simulink model "simRouteA_v4_11"  (R2015a)
settings: Solver=FixedStepDiscrete  StartTime=0.0  StopTime=36000  FixedStep=1  RelTol=1e-3
PreLoadFcn:
  | loadTimetable
StopFcn:
  | postProcess
undefined symbols (not defined in the file or in its folder): setBus1IntergenTime, setBus2IntergenTime, setBus3IntergenTime, setBus4IntergenTime
(part 1 of 7)
settings Model: Creator=nhuynh  LastModifiedBy=nhuynh
settings OptimizationCC: ExpressionDepthLimit=2147483647
settings DebuggingCC: UnderspecifiedInitializationDetection=Classic  MergeDetectMultiDrivingBlocksExec=none  SolverPrmCheckMsg=warning  StateNameClashWarn=warning

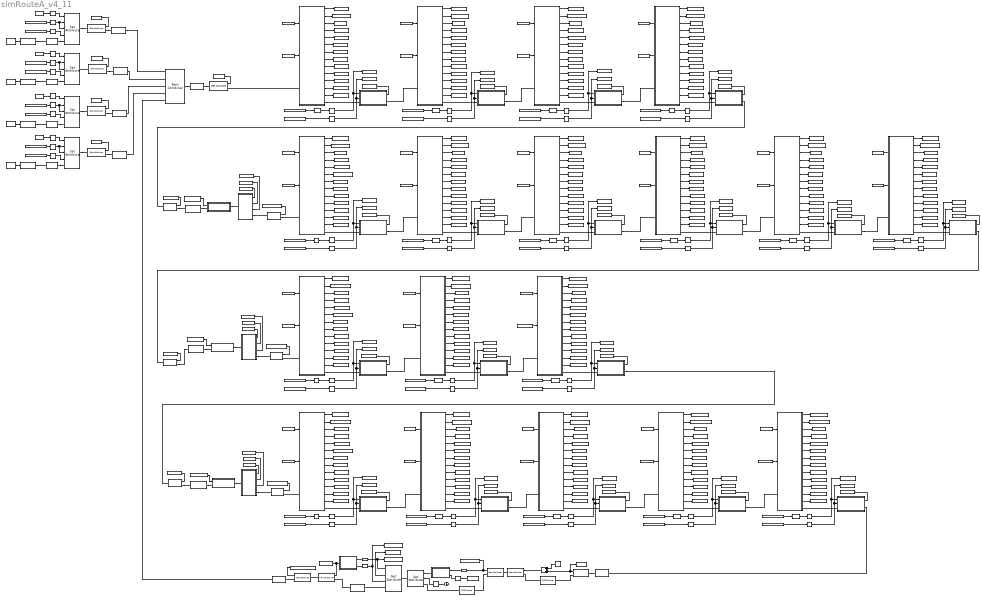
== system simRouteA_v4_11 ==
  Add : Sum
  Clock : Clock
  Constant : Constant
  Constant1 : Constant  Value=20000
  Constant2 : Constant  Value=10000
  Constant3 : Constant  Value=30000
  Constant4 : Constant  Value=40000
  Event Filter : EventFilter  ExecuteSubsystem=Upon sample time hit  SignalEdgeType=Rising
  Event Filter2 : EventFilter  ExecuteSubsystem=Upon sample time hit  SignalEdgeType=Rising
  Event Filter3 : EventFilter  ExecuteSubsystem=Upon sample time hit  SignalEdgeType=Rising
  FIFO Queue{2..6,8,10,13..17} (12 alike) : FIFOQueue
  From Workspace1 : FromWorkspace  VariableName=timetable  Interpolate=off  OutputAfterFinalValue=Holding final value
  From Workspace2 : FromWorkspace  VariableName=timetblChkPnt2  Interpolate=off  OutputAfterFinalValue=Holding final value
  From Workspace3 : FromWorkspace  VariableName=timetblChkPnt3  Interpolate=off  OutputAfterFinalValue=Holding final value
  From Workspace4 : FromWorkspace  VariableName=timetblChkPnt4  Interpolate=off  OutputAfterFinalValue=Holding final value
  Get Attribute{,2,4..8,10..13,17,19,22} (14 alike) : GetAttribute  AttributeName=ID  EvaluatedDefaultAttributeValue={ []}
      settings: OutputPortMap=o1
  Get Attribute3 : GetAttribute  AttributeName=tSched|ID|time  AttributeMissing=Error|Error|Error  AttributeDefaultValue=1|1|1  AttributeTreatAsVector=1|1|1  AttributeSendTiming=After entity departure|After entity departure|After entity departure  EvaluatedDefaultAttributeValue={ []; []; []}
      settings: OutputPortMap=o1,o2,o3
  HoldMultiBus : InfiniteServer  ServiceTimeFrom=Signal port t
  Path Combiner : PathCombiner  NumberInputPorts=5
  Rounding{,1..17} (18 alike) : Rounding  Operator=round
  Set Attribute{,3..5} (4 alike) : SetAttribute  AttributeName=ID|maxCap|vacancy|sec2Brd  AttributeFrom=Signal port|Signal port|Signal port|Signal port  AttributeValue=1|1|1|1  AttributeTreatAsVector=1|1|1|1  EvaluatedAttributeValue={ []; []; []; [] }
      settings: InputPortMap=u0,u1,u2,u3
  Set Attribute8 : SetAttribute  AttributeName=tSched|time  AttributeFrom=Signal port|Signal port  AttributeValue=1|1  AttributeTreatAsVector=1|1  EvaluatedAttributeValue={ []; [] }
      settings: InputPortMap=u0,u1
  Set Attribute9 : SetAttribute  AttributeName=ID  AttributeFrom=Signal port  EvaluatedAttributeValue={ [] }
  Subsystem : Subsystem  TreatAsAtomicUnit=on
      settings: MinAlgLoopOccurrences=on
  Subsystem3 : Subsystem  TreatAsAtomicUnit=on
  T2E{1,4..5,7..10,12..17,19..27,30..31,34..45,48..53,56..59,61..64} (50 alike) : TimedToEventSignal
  atStopS1 : Subsystem
  atStopS10 : Subsystem
  atStopS11 : Subsystem
  atStopS12 : Subsystem
  atStopS13 : Subsystem
  atStopS14 : Subsystem
  atStopS15 : Subsystem
  atStopS16 : Subsystem
  atStopS17 : Subsystem
  atStopS18 : Subsystem
  atStopS2 : Subsystem
  atStopS3 : Subsystem
  atStopS4 : Subsystem
  atStopS5 : Subsystem
  atStopS6 : Subsystem
  atStopS7 : Subsystem
  atStopS8 : Subsystem
  atStopS9 : Subsystem
  bus1Generator : TimeBasedEntityGenerator  GenerateEntitiesUpon=Intergeneration time from port t  GenerateEntityAtSimulationStart=off
  bus1IntergenTime : EventBasedSequence  VectorOutputValues=setBus1IntergenTime()  FormOutputOpt=Setting to infinity
  bus2Generator : TimeBasedEntityGenerator  GenerateEntitiesUpon=Intergeneration time from port t  GenerateEntityAtSimulationStart=off
  bus2IntergenTime : EventBasedSequence  VectorOutputValues=setBus2IntergenTime()  FormOutputOpt=Setting to infinity
  bus3Generator : TimeBasedEntityGenerator  GenerateEntitiesUpon=Intergeneration time from port t  GenerateEntityAtSimulationStart=off
  bus3IntergenTime : EventBasedSequence  VectorOutputValues=setBus3IntergenTime()  FormOutputOpt=Setting to infinity
  bus4Generator : TimeBasedEntityGenerator  GenerateEntitiesUpon=Intergeneration time from port t  GenerateEntityAtSimulationStart=off
  bus4IntergenTime : EventBasedSequence  VectorOutputValues=setBus4IntergenTime()  FormOutputOpt=Setting to infinity
  busIDOut : ToWorkspace  VariableName=busIDOut  SaveFormat=Structure With Time  SampleTime=-1
  chkSchedTimeNormalBusAtCP2 : Subsystem
  chkSchedTimeNormalBusAtCP3 : Subsystem
  chkSchedTimeNormalBusAtCP4 : Subsystem
  delayL1 : FromWorkspace  VariableName=[tLinkDelay,delayL1]  SampleTime=0  OutputAfterFinalValue=Setting to zero
  delayL10 : FromWorkspace  VariableName=[tLinkDelay,delayL10]  SampleTime=0  OutputAfterFinalValue=Setting to zero
  delayL11 : FromWorkspace  VariableName=[tLinkDelay,delayL11]  SampleTime=0  OutputAfterFinalValue=Setting to zero
  delayL12 : FromWorkspace  VariableName=[tLinkDelay,delayL12]  SampleTime=0  OutputAfterFinalValue=Setting to zero
  delayL13 : FromWorkspace  VariableName=[tLinkDelay,delayL13]  SampleTime=0  OutputAfterFinalValue=Setting to zero
  delayL14 : FromWorkspace  VariableName=[tLinkDelay,delayL14]  SampleTime=0  OutputAfterFinalValue=Setting to zero
  delayL15 : FromWorkspace  VariableName=[tLinkDelay,delayL15]  SampleTime=0  OutputAfterFinalValue=Setting to zero
  delayL16 : FromWorkspace  VariableName=[tLinkDelay,delayL16]  SampleTime=0  OutputAfterFinalValue=Setting to zero
  delayL17 : FromWorkspace  VariableName=[tLinkDelay,delayL17]  SampleTime=0  OutputAfterFinalValue=Setting to zero
  delayL18 : FromWorkspace  VariableName=[tLinkDelay,delayL18]  SampleTime=0  OutputAfterFinalValue=Setting to zero
  delayL2 : FromWorkspace  VariableName=[tLinkDelay,delayL2]  SampleTime=0  OutputAfterFinalValue=Setting to zero
  delayL3 : FromWorkspace  VariableName=[tLinkDelay,delayL3]  SampleTime=0  OutputAfterFinalValue=Setting to zero
  delayL4 : FromWorkspace  VariableName=[tLinkDelay,delayL4]  SampleTime=0  OutputAfterFinalValue=Setting to zero
  delayL5 : FromWorkspace  VariableName=[tLinkDelay,delayL5]  SampleTime=0  OutputAfterFinalValue=Setting to zero
  delayL6 : FromWorkspace  VariableName=[tLinkDelay,delayL6]  SampleTime=0  OutputAfterFinalValue=Setting to zero
  delayL7 : FromWorkspace  VariableName=[tLinkDelay,delayL7]  SampleTime=0  OutputAfterFinalValue=Setting to zero
  delayL8 : FromWorkspace  VariableName=[tLinkDelay,delayL8]  SampleTime=0  OutputAfterFinalValue=Setting to zero
  delayL9 : FromWorkspace  VariableName=[tLinkDelay,delayL9]  SampleTime=0  OutputAfterFinalValue=Setting to zero
  dummy Server{,1..3} (4 alike) : SingleServer  ServiceTime=0
  dummyServer : SingleServer  ServiceTime=0
  holdBusAtCP2 : Subsystem
  holdBusAtCP3 : Subsystem
  holdBusAtCP4 : Subsystem
  idAfterCycle : ToWorkspace  VariableName=idAfterCycle  SaveFormat=Structure With Time  SampleTime=-1
  idB4CP2 : ToWorkspace  VariableName=idB4CP2  SaveFormat=Structure With Time  SampleTime=-1
  idB4CP3 : ToWorkspace  VariableName=idB4CP3  SaveFormat=Structure With Time  SampleTime=-1
  idB4CP4 : ToWorkspace  VariableName=idB4CP4  SaveFormat=Structure With Time  SampleTime=-1
  idBus1SA : ToWorkspace  VariableName=idBus1SA  SaveFormat=Structure With Time  SampleTime=-1
  idBus2SA : ToWorkspace  VariableName=idBus2SA  SaveFormat=Structure With Time  SampleTime=-1
  idBus3SA : ToWorkspace  VariableName=idBus3SA  SaveFormat=Structure With Time  SampleTime=-1
  idBus4SA : ToWorkspace  VariableName=idBus4SA  SaveFormat=Structure With Time  SampleTime=-1
  idBusArrAfterCPS11 : ToWorkspace  VariableName=idBusArrAfterCPS11  SaveFormat=Structure With Time  SampleTime=-1
  idBusArrAfterCPS14 : ToWorkspace  VariableName=idBusArrAfterCPS14  SaveFormat=Structure With Time  SampleTime=-1
  idBusArrAfterCPS5 : ToWorkspace  VariableName=idBusArrAfterCPS5  SaveFormat=Structure With Time  SampleTime=-1
  idBusArrS1 : ToWorkspace  VariableName=idBusArrS1  SaveFormat=Structure With Time  SampleTime=-1
  idBusArrS10 : ToWorkspace  VariableName=idBusArrS10  SaveFormat=Structure With Time  SampleTime=-1
  idBusArrS11 : ToWorkspace  VariableName=idBusArrS11  SaveFormat=Structure With Time  SampleTime=-1
  idBusArrS12 : ToWorkspace  VariableName=idBusArrS12  SaveFormat=Structure With Time  SampleTime=-1
  idBusArrS13 : ToWorkspace  VariableName=idBusArrS13  SaveFormat=Structure With Time  SampleTime=-1
  idBusArrS14 : ToWorkspace  VariableName=idBusArrS14  SaveFormat=Structure With Time  SampleTime=-1
  idBusArrS15 : ToWorkspace  VariableName=idBusArrS15  SaveFormat=Structure With Time  SampleTime=-1
  idBusArrS16 : ToWorkspace  VariableName=idBusArrS16  SaveFormat=Structure With Time  SampleTime=-1
  idBusArrS17 : ToWorkspace  VariableName=idBusArrS17  SaveFormat=Structure With Time  SampleTime=-1
  idBusArrS18 : ToWorkspace  VariableName=idBusArrS18  SaveFormat=Structure With Time  SampleTime=-1
  idBusArrS2 : ToWorkspace  VariableName=idBusArrS2  SaveFormat=Structure With Time  SampleTime=-1
  idBusArrS3 : ToWorkspace  VariableName=idBusArrS3  SaveFormat=Structure With Time  SampleTime=-1
  idBusArrS4 : ToWorkspace  VariableName=idBusArrS4  SaveFormat=Structure With Time  SampleTime=-1
  idBusArrS5 : ToWorkspace  VariableName=idBusArrS5  SaveFormat=Structure With Time  SampleTime=-1
  idBusArrS6 : ToWorkspace  VariableName=idBusArrS6  SaveFormat=Structure With Time  SampleTime=-1
  idBusArrS7 : ToWorkspace  VariableName=idBusArrS7  SaveFormat=Structure With Time  SampleTime=-1
  idBusArrS8 : ToWorkspace  VariableName=idBusArrS8  SaveFormat=Structure With Time  SampleTime=-1
  idBusArrS9 : ToWorkspace  VariableName=idBusArrS9  SaveFormat=Structure With Time  SampleTime=-1
  idBusOutChkPntEndCycle : ToWorkspace  VariableName=idBusOutChkPntEndCycle  SaveFormat=Structure With Time  SampleTime=-1
  idBusOutChkPntS11 : ToWorkspace  VariableName=idBusOutChkPntS11  SaveFormat=Structure With Time  SampleTime=-1
  idBusOutChkPntS14 : ToWorkspace  VariableName=idBusOutChkPntS14  SaveFormat=Structure With Time  SampleTime=-1
  idBusOutChkPntS5 : ToWorkspace  VariableName=idBusOutChkPntS5  SaveFormat=Structure With Time  SampleTime=-1
  idBusOutL1 : ToWorkspace  VariableName=idBusOutL1  SaveFormat=Structure With Time  SampleTime=-1
  idBusOutL10 : ToWorkspace  VariableName=idBusOutL10  SaveFormat=Structure With Time  SampleTime=-1
  idBusOutL11 : ToWorkspace  VariableName=idBusOutL11  SaveFormat=Structure With Time  SampleTime=-1
  idBusOutL12 : ToWorkspace  VariableName=idBusOutL12  SaveFormat=Structure With Time  SampleTime=-1
  idBusOutL13 : ToWorkspace  VariableName=idBusOutL13  SaveFormat=Structure With Time  SampleTime=-1
  idBusOutL14 : ToWorkspace  VariableName=idBusOutL14  SaveFormat=Structure With Time  SampleTime=-1
  idBusOutL15 : ToWorkspace  VariableName=idBusOutL15  SaveFormat=Structure With Time  SampleTime=-1
  idBusOutL16 : ToWorkspace  VariableName=idBusOutL16  SaveFormat=Structure With Time  SampleTime=-1
  idBusOutL17 : ToWorkspace  VariableName=idBusOutL17  SaveFormat=Structure With Time  SampleTime=-1
  idBusOutL18 : ToWorkspace  VariableName=idBusOutL18  SaveFormat=Structure With Time  SampleTime=-1
  idBusOutL2 : ToWorkspace  VariableName=idBusOutL2  SaveFormat=Structure With Time  SampleTime=-1
  idBusOutL3 : ToWorkspace  VariableName=idBusOutL3  SaveFormat=Structure With Time  SampleTime=-1
  idBusOutL4 : ToWorkspace  VariableName=idBusOutL4  SaveFormat=Structure With Time  SampleTime=-1
  idBusOutL5 : ToWorkspace  VariableName=idBusOutL5  SaveFormat=Structure With Time  SampleTime=-1
  idBusOutL6 : ToWorkspace  VariableName=idBusOutL6  SaveFormat=Structure With Time  SampleTime=-1
  idBusOutL7 : ToWorkspace  VariableName=idBusOutL7  SaveFormat=Structure With Time  SampleTime=-1
  idBusOutL8 : ToWorkspace  VariableName=idBusOutL8  SaveFormat=Structure With Time  SampleTime=-1
  idBusOutL9 : ToWorkspace  VariableName=idBusOutL9  SaveFormat=Structure With Time  SampleTime=-1
  idBusOutS1 : ToWorkspace  VariableName=idBusOutS1  SaveFormat=Structure With Time  SampleTime=-1
  idBusOutS10 : ToWorkspace  VariableName=idBusOutS10  SaveFormat=Structure With Time  SampleTime=-1
  idBusOutS11 : ToWorkspace  VariableName=idBusOutS11  SaveFormat=Structure With Time  SampleTime=-1
  idBusOutS12 : ToWorkspace  VariableName=idBusOutS12  SaveFormat=Structure With Time  SampleTime=-1
  idBusOutS13 : ToWorkspace  VariableName=idBusOutS13  SaveFormat=Structure With Time  SampleTime=-1
  idBusOutS14 : ToWorkspace  VariableName=idBusOutS14  SaveFormat=Structure With Time  SampleTime=-1
  idBusOutS15 : ToWorkspace  VariableName=idBusOutS15  SaveFormat=Structure With Time  SampleTime=-1
  idBusOutS16 : ToWorkspace  VariableName=idBusOutS16  SaveFormat=Structure With Time  SampleTime=-1
  idBusOutS17 : ToWorkspace  VariableName=idBusOutS17  SaveFormat=Structure With Time  SampleTime=-1
  idBusOutS18 : ToWorkspace  VariableName=idBusOutS18  SaveFormat=Structure With Time  SampleTime=-1
  idBusOutS2 : ToWorkspace  VariableName=idBusOutS2  SaveFormat=Structure With Time  SampleTime=-1
  idBusOutS3 : ToWorkspace  VariableName=idBusOutS3  SaveFormat=Structure With Time  SampleTime=-1
  idBusOutS4 : ToWorkspace  VariableName=idBusOutS4  SaveFormat=Structure With Time  SampleTime=-1
  idBusOutS5 : ToWorkspace  VariableName=idBusOutS5  SaveFormat=Structure With Time  SampleTime=-1
  idBusOutS6 : ToWorkspace  VariableName=idBusOutS6  SaveFormat=Structure With Time  SampleTime=-1
  idBusOutS7 : ToWorkspace  VariableName=idBusOutS7  SaveFormat=Structure With Time  SampleTime=-1
  idBusOutS8 : ToWorkspace  VariableName=idBusOutS8  SaveFormat=Structure With Time  SampleTime=-1
  idBusOutS9 : ToWorkspace  VariableName=idBusOutS9  SaveFormat=Structure With Time  SampleTime=-1
  idInit : ToWorkspace  VariableName=idInit  SaveFormat=Structure With Time  SampleTime=-1
  idNxtNormalBus : ToWorkspace  VariableName=idNxtNormalBus  SaveFormat=Structure With Time  SampleTime=-1
  inTransitLinkL1 : Subsystem
  inTransitLinkL10 : Subsystem
  inTransitLinkL11 : Subsystem
  inTransitLinkL12 : Subsystem
  inTransitLinkL13 : Subsystem
  inTransitLinkL14 : Subsystem
  inTransitLinkL15 : Subsystem
  inTransitLinkL16 : Subsystem
  inTransitLinkL17 : Subsystem
  inTransitLinkL18 : Subsystem
  inTransitLinkL2 : Subsystem
  inTransitLinkL3 : Subsystem
  inTransitLinkL4 : Subsystem
  inTransitLinkL5 : Subsystem
  inTransitLinkL6 : Subsystem
  inTransitLinkL7 : Subsystem
  inTransitLinkL8 : Subsystem
  inTransitLinkL9 : Subsystem
  intgPaxAlightS1 : ToWorkspace  VariableName=paxAlightIntS1  SaveFormat=Structure With Time  SampleTime=-1
  intgPaxAlightS10 : ToWorkspace  VariableName=paxAlightIntS10  SaveFormat=Structure With Time  SampleTime=-1
  intgPaxAlightS11 : ToWorkspace  VariableName=paxAlightIntS11  SaveFormat=Structure With Time  SampleTime=-1
  intgPaxAlightS12 : ToWorkspace  VariableName=paxAlightIntS12  SaveFormat=Structure With Time  SampleTime=-1
  intgPaxAlightS13 : ToWorkspace  VariableName=paxAlightIntS13  SaveFormat=Structure With Time  SampleTime=-1
  intgPaxAlightS14 : ToWorkspace  VariableName=paxAlightIntS14  SaveFormat=Structure With Time  SampleTime=-1
  intgPaxAlightS15 : ToWorkspace  VariableName=paxAlightIntS15  SaveFormat=Structure With Time  SampleTime=-1
  intgPaxAlightS16 : ToWorkspace  VariableName=paxAlightIntS16  SaveFormat=Structure With Time  SampleTime=-1
  intgPaxAlightS17 : ToWorkspace  VariableName=paxAlightIntS17  SaveFormat=Structure With Time  SampleTime=-1
  intgPaxAlightS18 : ToWorkspace  VariableName=paxAlightIntS18  SaveFormat=Structure With Time  SampleTime=-1
  intgPaxAlightS2 : ToWorkspace  VariableName=paxAlightIntS2  SaveFormat=Structure With Time  SampleTime=-1
  intgPaxAlightS3 : ToWorkspace  VariableName=paxAlightIntS3  SaveFormat=Structure With Time  SampleTime=-1
  intgPaxAlightS4 : ToWorkspace  VariableName=paxAlightIntS4  SaveFormat=Structure With Time  SampleTime=-1
  intgPaxAlightS5 : ToWorkspace  VariableName=paxAlightIntS5  SaveFormat=Structure With Time  SampleTime=-1
  intgPaxAlightS6 : ToWorkspace  VariableName=paxAlightIntS6  SaveFormat=Structure With Time  SampleTime=-1
  intgPaxAlightS7 : ToWorkspace  VariableName=paxAlightIntS7  SaveFormat=Structure With Time  SampleTime=-1
  intgPaxAlightS8 : ToWorkspace  VariableName=paxAlightIntS8  SaveFormat=Structure With Time  SampleTime=-1
  intgPaxAlightS9 : ToWorkspace  VariableName=paxAlightIntS9  SaveFormat=Structure With Time  SampleTime=-1
  intgPaxArrS1 : ToWorkspace  VariableName=paxArrIntS1  SaveFormat=Structure With Time  SampleTime=-1
  intgPaxArrS10 : ToWorkspace  VariableName=paxArrIntS10  SaveFormat=Structure With Time  SampleTime=-1
  intgPaxArrS11 : ToWorkspace  VariableName=paxArrIntS11  SaveFormat=Structure With Time  SampleTime=-1
  intgPaxArrS12 : ToWorkspace  VariableName=paxArrIntS12  SaveFormat=Structure With Time  SampleTime=-1
  intgPaxArrS13 : ToWorkspace  VariableName=paxArrIntS13  SaveFormat=Structure With Time  SampleTime=-1
  intgPaxArrS14 : ToWorkspace  VariableName=paxArrIntS14  SaveFormat=Structure With Time  SampleTime=-1
  intgPaxArrS15 : ToWorkspace  VariableName=paxArrIntS15  SaveFormat=Structure With Time  SampleTime=-1
  intgPaxArrS16 : ToWorkspace  VariableName=paxArrIntS16  SaveFormat=Structure With Time  SampleTime=-1
  intgPaxArrS17 : ToWorkspace  VariableName=paxArrIntS17  SaveFormat=Structure With Time  SampleTime=-1
  intgPaxArrS18 : ToWorkspace  VariableName=paxArrIntS18  SaveFormat=Structure With Time  SampleTime=-1
  intgPaxArrS2 : ToWorkspace  VariableName=paxArrIntS2  SaveFormat=Structure With Time  SampleTime=-1
  intgPaxArrS3 : ToWorkspace  VariableName=paxArrIntS3  SaveFormat=Structure With Time  SampleTime=-1
  intgPaxArrS4 : ToWorkspace  VariableName=paxArrIntS4  SaveFormat=Structure With Time  SampleTime=-1
  intgPaxArrS5 : ToWorkspace  VariableName=paxArrIntS5  SaveFormat=Structure With Time  SampleTime=-1
  intgPaxArrS6 : ToWorkspace  VariableName=paxArrIntS6  SaveFormat=Structure With Time  SampleTime=-1
  intgPaxArrS7 : ToWorkspace  VariableName=paxArrIntS7  SaveFormat=Structure With Time  SampleTime=-1
  intgPaxArrS8 : ToWorkspace  VariableName=paxArrIntS8  SaveFormat=Structure With Time  SampleTime=-1
  intgPaxArrS9 : ToWorkspace  VariableName=paxArrIntS9  SaveFormat=Structure With Time  SampleTime=-1
  maxCapBus{1..4} (4 alike) : FromWorkspace  VariableName=[tConst,maxBusCap]  SampleTime=0  OutputAfterFinalValue=Holding final value
  newVacanS1 : ToWorkspace  VariableName=newVacanS1  SaveFormat=Structure With Time  SampleTime=-1
  newVacanS10 : ToWorkspace  VariableName=newVacanS10  SaveFormat=Structure With Time  SampleTime=-1
  newVacanS11 : ToWorkspace  VariableName=newVacanS11  SaveFormat=Structure With Time  SampleTime=-1
  newVacanS12 : ToWorkspace  VariableName=newVacanS12  SaveFormat=Structure With Time  SampleTime=-1
  newVacanS13 : ToWorkspace  VariableName=newVacanS13  SaveFormat=Structure With Time  SampleTime=-1
  newVacanS14 : ToWorkspace  VariableName=newVacanS14  SaveFormat=Structure With Time  SampleTime=-1
  newVacanS15 : ToWorkspace  VariableName=newVacanS15  SaveFormat=Structure With Time  SampleTime=-1
  newVacanS16 : ToWorkspace  VariableName=newVacanS16  SaveFormat=Structure With Time  SampleTime=-1
  newVacanS17 : ToWorkspace  VariableName=newVacanS17  SaveFormat=Structure With Time  SampleTime=-1
  newVacanS18 : ToWorkspace  VariableName=newVacanS18  SaveFormat=Structure With Time  SampleTime=-1
  newVacanS2 : ToWorkspace  VariableName=newVacanS2  SaveFormat=Structure With Time  SampleTime=-1
  newVacanS3 : ToWorkspace  VariableName=newVacanS3  SaveFormat=Structure With Time  SampleTime=-1
  newVacanS4 : ToWorkspace  VariableName=newVacanS4  SaveFormat=Structure With Time  SampleTime=-1
  newVacanS5 : ToWorkspace  VariableName=newVacanS5  SaveFormat=Structure With Time  SampleTime=-1
  newVacanS6 : ToWorkspace  VariableName=newVacanS6  SaveFormat=Structure With Time  SampleTime=-1
  newVacanS7 : ToWorkspace  VariableName=newVacanS7  SaveFormat=Structure With Time  SampleTime=-1
  newVacanS8 : ToWorkspace  VariableName=newVacanS8  SaveFormat=Structure With Time  SampleTime=-1
  newVacanS9 : ToWorkspace  VariableName=newVacanS9  SaveFormat=Structure With Time  SampleTime=-1
  paxAlightS1 : ToWorkspace  VariableName=paxAlightS1  SaveFormat=Structure With Time  SampleTime=-1
  paxAlightS10 : ToWorkspace  VariableName=paxAlightS10  SaveFormat=Structure With Time  SampleTime=-1
  paxAlightS11 : ToWorkspace  VariableName=paxAlightS11  SaveFormat=Structure With Time  SampleTime=-1
  paxAlightS12 : ToWorkspace  VariableName=paxAlightS12  SaveFormat=Structure With Time  SampleTime=-1
  paxAlightS13 : ToWorkspace  VariableName=paxAlightS13  SaveFormat=Structure With Time  SampleTime=-1
  paxAlightS14 : ToWorkspace  VariableName=paxAlightS14  SaveFormat=Structure With Time  SampleTime=-1
  paxAlightS15 : ToWorkspace  VariableName=paxAlightS15  SaveFormat=Structure With Time  SampleTime=-1
  paxAlightS16 : ToWorkspace  VariableName=paxAlightS16  SaveFormat=Structure With Time  SampleTime=-1
  paxAlightS17 : ToWorkspace  VariableName=paxAlightS17  SaveFormat=Structure With Time  SampleTime=-1
  paxAlightS18 : ToWorkspace  VariableName=paxAlightS18  SaveFormat=Structure With Time  SampleTime=-1
  paxAlightS2 : ToWorkspace  VariableName=paxAlightS2  SaveFormat=Structure With Time  SampleTime=-1
  paxAlightS3 : ToWorkspace  VariableName=paxAlightS3  SaveFormat=Structure With Time  SampleTime=-1
  paxAlightS4 : ToWorkspace  VariableName=paxAlightS4  SaveFormat=Structure With Time  SampleTime=-1
  paxAlightS5 : ToWorkspace  VariableName=paxAlightS5  SaveFormat=Structure With Time  SampleTime=-1
  paxAlightS6 : ToWorkspace  VariableName=paxAlightS6  SaveFormat=Structure With Time  SampleTime=-1
  paxAlightS7 : ToWorkspace  VariableName=paxAlightS7  SaveFormat=Structure With Time  SampleTime=-1
  paxAlightS8 : ToWorkspace  VariableName=paxAlightS8  SaveFormat=Structure With Time  SampleTime=-1
  paxAlightS9 : ToWorkspace  VariableName=paxAlightS9  SaveFormat=Structure With Time  SampleTime=-1
  paxBoardS1 : ToWorkspace  VariableName=paxBoardS1  SaveFormat=Structure With Time  SampleTime=-1
  paxBoardS10 : ToWorkspace  VariableName=paxBoardS10  SaveFormat=Structure With Time  SampleTime=-1
  paxBoardS11 : ToWorkspace  VariableName=paxBoardS11  SaveFormat=Structure With Time  SampleTime=-1
  paxBoardS12 : ToWorkspace  VariableName=paxBoardS12  SaveFormat=Structure With Time  SampleTime=-1
  paxBoardS13 : ToWorkspace  VariableName=paxBoardS13  SaveFormat=Structure With Time  SampleTime=-1
  paxBoardS14 : ToWorkspace  VariableName=paxBoardS14  SaveFormat=Structure With Time  SampleTime=-1
  paxBoardS15 : ToWorkspace  VariableName=paxBoardS15  SaveFormat=Structure With Time  SampleTime=-1
  paxBoardS16 : ToWorkspace  VariableName=paxBoardS16  SaveFormat=Structure With Time  SampleTime=-1
  paxBoardS17 : ToWorkspace  VariableName=paxBoardS17  SaveFormat=Structure With Time  SampleTime=-1
  paxBoardS18 : ToWorkspace  VariableName=paxBoardS18  SaveFormat=Structure With Time  SampleTime=-1
  paxBoardS2 : ToWorkspace  VariableName=paxBoardS2  SaveFormat=Structure With Time  SampleTime=-1
  paxBoardS3 : ToWorkspace  VariableName=paxBoardS3  SaveFormat=Structure With Time  SampleTime=-1
  paxBoardS4 : ToWorkspace  VariableName=paxBoardS4  SaveFormat=Structure With Time  SampleTime=-1
  paxBoardS5 : ToWorkspace  VariableName=paxBoardS5  SaveFormat=Structure With Time  SampleTime=-1
  paxBoardS6 : ToWorkspace  VariableName=paxBoardS6  SaveFormat=Structure With Time  SampleTime=-1
  paxBoardS7 : ToWorkspace  VariableName=paxBoardS7  SaveFormat=Structure With Time  SampleTime=-1
  paxBoardS8 : ToWorkspace  VariableName=paxBoardS8  SaveFormat=Structure With Time  SampleTime=-1
  paxBoardS9 : ToWorkspace  VariableName=paxBoardS9  SaveFormat=Structure With Time  SampleTime=-1
  paxDemandS1 : ToWorkspace  VariableName=paxDemandS1  SaveFormat=Structure With Time  SampleTime=-1
  paxDemandS10 : ToWorkspace  VariableName=paxDemandS10  SaveFormat=Structure With Time  SampleTime=-1
  paxDemandS11 : ToWorkspace  VariableName=paxDemandS11  SaveFormat=Structure With Time  SampleTime=-1
  paxDemandS12 : ToWorkspace  VariableName=paxDemandS12  SaveFormat=Structure With Time  SampleTime=-1
  paxDemandS13 : ToWorkspace  VariableName=paxDemandS13  SaveFormat=Structure With Time  SampleTime=-1
  paxDemandS14 : ToWorkspace  VariableName=paxDemandS14  SaveFormat=Structure With Time  SampleTime=-1
  paxDemandS15 : ToWorkspace  VariableName=paxDemandS15  SaveFormat=Structure With Time  SampleTime=-1
  paxDemandS16 : ToWorkspace  VariableName=paxDemandS16  SaveFormat=Structure With Time  SampleTime=-1
  paxDemandS17 : ToWorkspace  VariableName=paxDemandS17  SaveFormat=Structure With Time  SampleTime=-1
  paxDemandS18 : ToWorkspace  VariableName=paxDemandS18  SaveFormat=Structure With Time  SampleTime=-1
  paxDemandS2 : ToWorkspace  VariableName=paxDemandS2  SaveFormat=Structure With Time  SampleTime=-1
  paxDemandS3 : ToWorkspace  VariableName=paxDemandS3  SaveFormat=Structure With Time  SampleTime=-1
  paxDemandS4 : ToWorkspace  VariableName=paxDemandS4  SaveFormat=Structure With Time  SampleTime=-1
  paxDemandS5 : ToWorkspace  VariableName=paxDemandS5  SaveFormat=Structure With Time  SampleTime=-1
  paxDemandS6 : ToWorkspace  VariableName=paxDemandS6  SaveFormat=Structure With Time  SampleTime=-1
  paxDemandS7 : ToWorkspace  VariableName=paxDemandS7  SaveFormat=Structure With Time  SampleTime=-1
  paxDemandS8 : ToWorkspace  VariableName=paxDemandS8  SaveFormat=Structure With Time  SampleTime=-1
  paxDemandS9 : ToWorkspace  VariableName=paxDemandS9  SaveFormat=Structure With Time  SampleTime=-1
  paxRemainS1 : ToWorkspace  VariableName=paxRemainS1  SaveFormat=Structure With Time  SampleTime=-1
  paxRemainS10 : ToWorkspace  VariableName=paxRemainS10  SaveFormat=Structure With Time  SampleTime=-1
  paxRemainS11 : ToWorkspace  VariableName=paxRemainS11  SaveFormat=Structure With Time  SampleTime=-1
  paxRemainS12 : ToWorkspace  VariableName=paxRemainS12  SaveFormat=Structure With Time  SampleTime=-1
  paxRemainS13 : ToWorkspace  VariableName=paxRemainS13  SaveFormat=Structure With Time  SampleTime=-1
  paxRemainS14 : ToWorkspace  VariableName=paxRemainS14  SaveFormat=Structure With Time  SampleTime=-1
  paxRemainS15 : ToWorkspace  VariableName=paxRemainS15  SaveFormat=Structure With Time  SampleTime=-1
  paxRemainS16 : ToWorkspace  VariableName=paxRemainS16  SaveFormat=Structure With Time  SampleTime=-1
  paxRemainS17 : ToWorkspace  VariableName=paxRemainS17  SaveFormat=Structure With Time  SampleTime=-1
  paxRemainS18 : ToWorkspace  VariableName=paxRemainS18  SaveFormat=Structure With Time  SampleTime=-1
  paxRemainS2 : ToWorkspace  VariableName=paxRemainS2  SaveFormat=Structure With Time  SampleTime=-1
  paxRemainS3 : ToWorkspace  VariableName=paxRemainS3  SaveFormat=Structure With Time  SampleTime=-1
  paxRemainS4 : ToWorkspace  VariableName=paxRemainS4  SaveFormat=Structure With Time  SampleTime=-1
  paxRemainS5 : ToWorkspace  VariableName=paxRemainS5  SaveFormat=Structure With Time  SampleTime=-1
  paxRemainS6 : ToWorkspace  VariableName=paxRemainS6  SaveFormat=Structure With Time  SampleTime=-1
  paxRemainS7 : ToWorkspace  VariableName=paxRemainS7  SaveFormat=Structure With Time  SampleTime=-1
  paxRemainS8 : ToWorkspace  VariableName=paxRemainS8  SaveFormat=Structure With Time  SampleTime=-1
  paxRemainS9 : ToWorkspace  VariableName=paxRemainS9  SaveFormat=Structure With Time  SampleTime=-1
  paxWaitS1 : ToWorkspace  VariableName=paxWaitS1  SaveFormat=Structure With Time  SampleTime=-1
  paxWaitS10 : ToWorkspace  VariableName=paxWaitS10  SaveFormat=Structure With Time  SampleTime=-1
  paxWaitS11 : ToWorkspace  VariableName=paxWaitS11  SaveFormat=Structure With Time  SampleTime=-1
  paxWaitS12 : ToWorkspace  VariableName=paxWaitS12  SaveFormat=Structure With Time  SampleTime=-1
  paxWaitS13 : ToWorkspace  VariableName=paxWaitS13  SaveFormat=Structure With Time  SampleTime=-1
  paxWaitS14 : ToWorkspace  VariableName=paxWaitS14  SaveFormat=Structure With Time  SampleTime=-1
  paxWaitS15 : ToWorkspace  VariableName=paxWaitS15  SaveFormat=Structure With Time  SampleTime=-1
  paxWaitS16 : ToWorkspace  VariableName=paxWaitS16  SaveFormat=Structure With Time  SampleTime=-1
  paxWaitS17 : ToWorkspace  VariableName=paxWaitS17  SaveFormat=Structure With Time  SampleTime=-1
  paxWaitS18 : ToWorkspace  VariableName=paxWaitS18  SaveFormat=Structure With Time  SampleTime=-1
  paxWaitS2 : ToWorkspace  VariableName=paxWaitS2  SaveFormat=Structure With Time  SampleTime=-1
  paxWaitS3 : ToWorkspace  VariableName=paxWaitS3  SaveFormat=Structure With Time  SampleTime=-1
  paxWaitS4 : ToWorkspace  VariableName=paxWaitS4  SaveFormat=Structure With Time  SampleTime=-1
  paxWaitS5 : ToWorkspace  VariableName=paxWaitS5  SaveFormat=Structure With Time  SampleTime=-1
  paxWaitS6 : ToWorkspace  VariableName=paxWaitS6  SaveFormat=Structure With Time  SampleTime=-1
  paxWaitS7 : ToWorkspace  VariableName=paxWaitS7  SaveFormat=Structure With Time  SampleTime=-1
  paxWaitS8 : ToWorkspace  VariableName=paxWaitS8  SaveFormat=Structure With Time  SampleTime=-1
  paxWaitS9 : ToWorkspace  VariableName=paxWaitS9  SaveFormat=Structure With Time  SampleTime=-1
  randDelayL1 : ToWorkspace  VariableName=randDelayL1  SaveFormat=Structure With Time  SampleTime=-1
  randDelayL10 : ToWorkspace  VariableName=randDelayL10  SaveFormat=Structure With Time  SampleTime=-1
  randDelayL11 : ToWorkspace  VariableName=randDelayL11  SaveFormat=Structure With Time  SampleTime=-1
  randDelayL12 : ToWorkspace  VariableName=randDelayL12  SaveFormat=Structure With Time  SampleTime=-1
  randDelayL13 : ToWorkspace  VariableName=randDelayL13  SaveFormat=Structure With Time  SampleTime=-1
  randDelayL14 : ToWorkspace  VariableName=randDelayL14  SaveFormat=Structure With Time  SampleTime=-1
  randDelayL15 : ToWorkspace  VariableName=randDelayL15  SaveFormat=Structure With Time  SampleTime=-1
  randDelayL16 : ToWorkspace  VariableName=randDelayL16  SaveFormat=Structure With Time  SampleTime=-1
  randDelayL17 : ToWorkspace  VariableName=randDelayL17  SaveFormat=Structure With Time  SampleTime=-1
  randDelayL18 : ToWorkspace  VariableName=randDelayL18  SaveFormat=Structure With Time  SampleTime=-1
  randDelayL2 : ToWorkspace  VariableName=randDelayL2  SaveFormat=Structure With Time  SampleTime=-1
  randDelayL3 : ToWorkspace  VariableName=randDelayL3  SaveFormat=Structure With Time  SampleTime=-1
  randDelayL4 : ToWorkspace  VariableName=randDelayL4  SaveFormat=Structure With Time  SampleTime=-1
  randDelayL5 : ToWorkspace  VariableName=randDelayL5  SaveFormat=Structure With Time  SampleTime=-1
  randDelayL6 : ToWorkspace  VariableName=randDelayL6  SaveFormat=Structure With Time  SampleTime=-1
  randDelayL7 : ToWorkspace  VariableName=randDelayL7  SaveFormat=Structure With Time  SampleTime=-1
  randDelayL8 : ToWorkspace  VariableName=randDelayL8  SaveFormat=Structure With Time  SampleTime=-1
  randDelayL9 : ToWorkspace  VariableName=randDelayL9  SaveFormat=Structure With Time  SampleTime=-1
  ratePaxAlightS1 : FromWorkspace  VariableName=[t,alightS1]  SampleTime=0  OutputAfterFinalValue=Setting to zero
  ratePaxAlightS10 : FromWorkspace  VariableName=[t,alightS10]  SampleTime=0  OutputAfterFinalValue=Setting to zero
  ratePaxAlightS11 : FromWorkspace  VariableName=[t,alightS11]  SampleTime=0  OutputAfterFinalValue=Setting to zero
  ratePaxAlightS12 : FromWorkspace  VariableName=[t,alightS12]  SampleTime=0  OutputAfterFinalValue=Setting to zero
  ratePaxAlightS13 : FromWorkspace  VariableName=[t,alightS13]  SampleTime=0  OutputAfterFinalValue=Setting to zero
  ratePaxAlightS14 : FromWorkspace  VariableName=[t,alightS14]  SampleTime=0  OutputAfterFinalValue=Setting to zero
  ratePaxAlightS15 : FromWorkspace  VariableName=[t,alightS15]  SampleTime=0  OutputAfterFinalValue=Setting to zero
  ratePaxAlightS16 : FromWorkspace  VariableName=[t,alightS16]  SampleTime=0  OutputAfterFinalValue=Setting to zero
  ratePaxAlightS17 : FromWorkspace  VariableName=[t,alightS17]  SampleTime=0  OutputAfterFinalValue=Setting to zero
  ratePaxAlightS18 : FromWorkspace  VariableName=[t,alightS18]  SampleTime=0  OutputAfterFinalValue=Setting to zero
  ratePaxAlightS2 : FromWorkspace  VariableName=[t,alightS2]  SampleTime=0  OutputAfterFinalValue=Setting to zero
  ratePaxAlightS3 : FromWorkspace  VariableName=[t,alightS3]  SampleTime=0  OutputAfterFinalValue=Setting to zero
  ratePaxAlightS4 : FromWorkspace  VariableName=[t,alightS4]  SampleTime=0  OutputAfterFinalValue=Setting to zero
  ratePaxAlightS5 : FromWorkspace  VariableName=[t,alightS5]  SampleTime=0  OutputAfterFinalValue=Setting to zero
  ratePaxAlightS6 : FromWorkspace  VariableName=[t,alightS6]  SampleTime=0  OutputAfterFinalValue=Setting to zero
  ratePaxAlightS7 : FromWorkspace  VariableName=[t,alightS7]  SampleTime=0  OutputAfterFinalValue=Setting to zero
  ratePaxAlightS8 : FromWorkspace  VariableName=[t,alightS8]  SampleTime=0  OutputAfterFinalValue=Setting to zero
  ratePaxAlightS9 : FromWorkspace  VariableName=[t,alightS9]  SampleTime=0  OutputAfterFinalValue=Setting to zero
  ratePaxArrS1 : FromWorkspace  VariableName=[t,arrS1]  SampleTime=0  OutputAfterFinalValue=Setting to zero
  ratePaxArrS10 : FromWorkspace  VariableName=[t,arrS10]  SampleTime=0  OutputAfterFinalValue=Setting to zero
  ratePaxArrS11 : FromWorkspace  VariableName=[t,arrS11]  SampleTime=0  OutputAfterFinalValue=Setting to zero
  ratePaxArrS12 : FromWorkspace  VariableName=[t,arrS12]  SampleTime=0  OutputAfterFinalValue=Setting to zero
  ratePaxArrS13 : FromWorkspace  VariableName=[t,arrS13]  SampleTime=0  OutputAfterFinalValue=Setting to zero
  ratePaxArrS14 : FromWorkspace  VariableName=[t,arrS14]  SampleTime=0  OutputAfterFinalValue=Setting to zero
  ratePaxArrS15 : FromWorkspace  VariableName=[t,arrS15]  SampleTime=0  OutputAfterFinalValue=Setting to zero
  ratePaxArrS16 : FromWorkspace  VariableName=[t,arrS16]  SampleTime=0  OutputAfterFinalValue=Setting to zero
  ratePaxArrS17 : FromWorkspace  VariableName=[t,arrS17]  SampleTime=0  OutputAfterFinalValue=Setting to zero
  ratePaxArrS18 : FromWorkspace  VariableName=[t,arrS18]  SampleTime=0  OutputAfterFinalValue=Setting to zero
  ratePaxArrS2 : FromWorkspace  VariableName=[t,arrS2]  SampleTime=0  OutputAfterFinalValue=Setting to zero
  ratePaxArrS3 : FromWorkspace  VariableName=[t,arrS3]  SampleTime=0  OutputAfterFinalValue=Setting to zero
  ratePaxArrS4 : FromWorkspace  VariableName=[t,arrS4]  SampleTime=0  OutputAfterFinalValue=Setting to zero
  ratePaxArrS5 : FromWorkspace  VariableName=[t,arrS5]  SampleTime=0  OutputAfterFinalValue=Setting to zero
  ratePaxArrS6 : FromWorkspace  VariableName=[t,arrS6]  SampleTime=0  OutputAfterFinalValue=Setting to zero
  ratePaxArrS7 : FromWorkspace  VariableName=[t,arrS7]  SampleTime=0  OutputAfterFinalValue=Setting to zero
  ratePaxArrS8 : FromWorkspace  VariableName=[t,arrS8]  SampleTime=0  OutputAfterFinalValue=Setting to zero
  ratePaxArrS9 : FromWorkspace  VariableName=[t,arrS9]  SampleTime=0  OutputAfterFinalValue=Setting to zero
  rawPaxAlightS1 : ToWorkspace  VariableName=rawPaxAlightS1  SaveFormat=Structure With Time  SampleTime=-1
  rawPaxAlightS10 : ToWorkspace  VariableName=rawPaxAlightS10  SaveFormat=Structure With Time  SampleTime=-1
  rawPaxAlightS11 : ToWorkspace  VariableName=rawPaxAlightS11  SaveFormat=Structure With Time  SampleTime=-1
  rawPaxAlightS12 : ToWorkspace  VariableName=rawPaxAlightS12  SaveFormat=Structure With Time  SampleTime=-1
  rawPaxAlightS13 : ToWorkspace  VariableName=rawPaxAlightS13  SaveFormat=Structure With Time  SampleTime=-1
  rawPaxAlightS14 : ToWorkspace  VariableName=rawPaxAlightS14  SaveFormat=Structure With Time  SampleTime=-1
  rawPaxAlightS15 : ToWorkspace  VariableName=rawPaxAlightS15  SaveFormat=Structure With Time  SampleTime=-1
  rawPaxAlightS16 : ToWorkspace  VariableName=rawPaxAlightS16  SaveFormat=Structure With Time  SampleTime=-1
  rawPaxAlightS17 : ToWorkspace  VariableName=rawPaxAlightS17  SaveFormat=Structure With Time  SampleTime=-1
  rawPaxAlightS18 : ToWorkspace  VariableName=rawPaxAlightS18  SaveFormat=Structure With Time  SampleTime=-1
  rawPaxAlightS2 : ToWorkspace  VariableName=rawPaxAlightS2  SaveFormat=Structure With Time  SampleTime=-1
  rawPaxAlightS3 : ToWorkspace  VariableName=rawPaxAlightS3  SaveFormat=Structure With Time  SampleTime=-1
  rawPaxAlightS4 : ToWorkspace  VariableName=rawPaxAlightS4  SaveFormat=Structure With Time  SampleTime=-1
  rawPaxAlightS5 : ToWorkspace  VariableName=rawPaxAlightS5  SaveFormat=Structure With Time  SampleTime=-1
  rawPaxAlightS6 : ToWorkspace  VariableName=rawPaxAlightS6  SaveFormat=Structure With Time  SampleTime=-1
  rawPaxAlightS7 : ToWorkspace  VariableName=rawPaxAlightS7  SaveFormat=Structure With Time  SampleTime=-1
  rawPaxAlightS8 : ToWorkspace  VariableName=rawPaxAlightS8  SaveFormat=Structure With Time  SampleTime=-1
  rawPaxAlightS9 : ToWorkspace  VariableName=rawPaxAlightS9  SaveFormat=Structure With Time  SampleTime=-1
  rawPaxDemandS1 : ToWorkspace  VariableName=rawPaxDemandS1  SaveFormat=Structure With Time  SampleTime=-1
  rawPaxDemandS10 : ToWorkspace  VariableName=rawPaxDemandS10  SaveFormat=Structure With Time  SampleTime=-1
  rawPaxDemandS11 : ToWorkspace  VariableName=rawPaxDemandS11  SaveFormat=Structure With Time  SampleTime=-1
  rawPaxDemandS12 : ToWorkspace  VariableName=rawPaxDemandS12  SaveFormat=Structure With Time  SampleTime=-1
  rawPaxDemandS13 : ToWorkspace  VariableName=rawPaxDemandS13  SaveFormat=Structure With Time  SampleTime=-1
  rawPaxDemandS14 : ToWorkspace  VariableName=rawPaxDemandS14  SaveFormat=Structure With Time  SampleTime=-1
  rawPaxDemandS15 : ToWorkspace  VariableName=rawPaxDemandS15  SaveFormat=Structure With Time  SampleTime=-1
  rawPaxDemandS16 : ToWorkspace  VariableName=rawPaxDemandS16  SaveFormat=Structure With Time  SampleTime=-1
  rawPaxDemandS17 : ToWorkspace  VariableName=rawPaxDemandS17  SaveFormat=Structure With Time  SampleTime=-1
  rawPaxDemandS18 : ToWorkspace  VariableName=rawPaxDemandS18  SaveFormat=Structure With Time  SampleTime=-1
  rawPaxDemandS2 : ToWorkspace  VariableName=rawPaxDemandS2  SaveFormat=Structure With Time  SampleTime=-1
  rawPaxDemandS3 : ToWorkspace  VariableName=rawPaxDemandS3  SaveFormat=Structure With Time  SampleTime=-1
  rawPaxDemandS4 : ToWorkspace  VariableName=rawPaxDemandS4  SaveFormat=Structure With Time  SampleTime=-1
  rawPaxDemandS5 : ToWorkspace  VariableName=rawPaxDemandS5  SaveFormat=Structure With Time  SampleTime=-1
  rawPaxDemandS6 : ToWorkspace  VariableName=rawPaxDemandS6  SaveFormat=Structure With Time  SampleTime=-1
  rawPaxDemandS7 : ToWorkspace  VariableName=rawPaxDemandS7  SaveFormat=Structure With Time  SampleTime=-1
  rawPaxDemandS8 : ToWorkspace  VariableName=rawPaxDemandS8  SaveFormat=Structure With Time  SampleTime=-1
  rawPaxDemandS9 : ToWorkspace  VariableName=rawPaxDemandS9  SaveFormat=Structure With Time  SampleTime=-1
  tBoardPerPax{,1..3} (4 alike) : FromWorkspace  VariableName=[tConst,tBoardPerPax]  SampleTime=0  OutputAfterFinalValue=Holding final value
  tHold : ToWorkspace  VariableName=tHold  SaveFormat=Structure With Time  SampleTime=-1
  tHoldCP2 : ToWorkspace  VariableName=tHoldCP2  SaveFormat=Structure With Time  SampleTime=-1
  tHoldCP3 : ToWorkspace  VariableName=tHoldCP3  SaveFormat=Structure With Time  SampleTime=-1
  tHoldCP4 : ToWorkspace  VariableName=tHoldCP4  SaveFormat=Structure With Time  SampleTime=-1
  tSchedCP2 : ToWorkspace  VariableName=tSchedCP2  SaveFormat=Structure With Time  SampleTime=-1
  tSchedCP3 : ToWorkspace  VariableName=tSchedCP3  SaveFormat=Structure With Time  SampleTime=-1
  tSchedCP4 : ToWorkspace  VariableName=tSchedCP4  SaveFormat=Structure With Time  SampleTime=-1
  tTravL1 : FromWorkspace  VariableName=[tTravTime,tTravL1]  SampleTime=0  OutputAfterFinalValue=Holding final value
  tTravL10 : FromWorkspace  VariableName=[tTravTime,tTravL10]  SampleTime=0  OutputAfterFinalValue=Holding final value
  tTravL11 : FromWorkspace  VariableName=[tTravTime,tTravL11]  SampleTime=0  OutputAfterFinalValue=Holding final value
  tTravL12 : FromWorkspace  VariableName=[tTravTime,tTravL12]  SampleTime=0  OutputAfterFinalValue=Holding final value
  tTravL13 : FromWorkspace  VariableName=[tTravTime,tTravL13]  SampleTime=0  OutputAfterFinalValue=Holding final value
  tTravL14 : FromWorkspace  VariableName=[tTravTime,tTravL14]  SampleTime=0  OutputAfterFinalValue=Holding final value
  tTravL15 : FromWorkspace  VariableName=[tTravTime,tTravL15]  SampleTime=0  OutputAfterFinalValue=Holding final value
  tTravL16 : FromWorkspace  VariableName=[tTravTime,tTravL16]  SampleTime=0  OutputAfterFinalValue=Holding final value
  tTravL17 : FromWorkspace  VariableName=[tTravTime,tTravL17]  SampleTime=0  OutputAfterFinalValue=Holding final value
  tTravL18 : FromWorkspace  VariableName=[tTravTime,tTravL18]  SampleTime=0  OutputAfterFinalValue=Holding final value
  tTravL2 : FromWorkspace  VariableName=[tTravTime,tTravL2]  SampleTime=0  OutputAfterFinalValue=Holding final value
  tTravL3 : FromWorkspace  VariableName=[tTravTime,tTravL3]  SampleTime=0  OutputAfterFinalValue=Holding final value
  tTravL4 : FromWorkspace  VariableName=[tTravTime,tTravL4]  SampleTime=0  OutputAfterFinalValue=Holding final value
  tTravL5 : FromWorkspace  VariableName=[tTravTime,tTravL5]  SampleTime=0  OutputAfterFinalValue=Holding final value
  tTravL6 : FromWorkspace  VariableName=[tTravTime,tTravL6]  SampleTime=0  OutputAfterFinalValue=Holding final value
  tTravL7 : FromWorkspace  VariableName=[tTravTime,tTravL7]  SampleTime=0  OutputAfterFinalValue=Holding final value
  tTravL8 : FromWorkspace  VariableName=[tTravTime,tTravL8]  SampleTime=0  OutputAfterFinalValue=Holding final value
  tTravL9 : FromWorkspace  VariableName=[tTravTime,tTravL9]  SampleTime=0  OutputAfterFinalValue=Holding final value
  timeArr : ToWorkspace  VariableName=timeArr  SaveFormat=Structure With Time  SampleTime=-1
  timeScheduled : ToWorkspace  VariableName=timeScheduled  SaveFormat=Structure With Time  SampleTime=-1
  travTimeL1 : ToWorkspace  VariableName=travTimeL1  SaveFormat=Structure With Time  SampleTime=-1
  travTimeL10 : ToWorkspace  VariableName=travTimeL10  SaveFormat=Structure With Time  SampleTime=-1
  travTimeL11 : ToWorkspace  VariableName=travTimeL11  SaveFormat=Structure With Time  SampleTime=-1
  travTimeL12 : ToWorkspace  VariableName=travTimeL12  SaveFormat=Structure With Time  SampleTime=-1
  travTimeL13 : ToWorkspace  VariableName=travTimeL13  SaveFormat=Structure With Time  SampleTime=-1
  travTimeL14 : ToWorkspace  VariableName=travTimeL14  SaveFormat=Structure With Time  SampleTime=-1
  travTimeL15 : ToWorkspace  VariableName=travTimeL15  SaveFormat=Structure With Time  SampleTime=-1
  travTimeL16 : ToWorkspace  VariableName=travTimeL16  SaveFormat=Structure With Time  SampleTime=-1
  travTimeL17 : ToWorkspace  VariableName=travTimeL17  SaveFormat=Structure With Time  SampleTime=-1
  travTimeL18 : ToWorkspace  VariableName=travTimeL18  SaveFormat=Structure With Time  SampleTime=-1
  travTimeL2 : ToWorkspace  VariableName=travTimeL2  SaveFormat=Structure With Time  SampleTime=-1
  travTimeL3 : ToWorkspace  VariableName=travTimeL3  SaveFormat=Structure With Time  SampleTime=-1
  travTimeL4 : ToWorkspace  VariableName=travTimeL4  SaveFormat=Structure With Time  SampleTime=-1
  travTimeL5 : ToWorkspace  VariableName=travTimeL5  SaveFormat=Structure With Time  SampleTime=-1
  travTimeL6 : ToWorkspace  VariableName=travTimeL6  SaveFormat=Structure With Time  SampleTime=-1
  travTimeL7 : ToWorkspace  VariableName=travTimeL7  SaveFormat=Structure With Time  SampleTime=-1
  travTimeL8 : ToWorkspace  VariableName=travTimeL8  SaveFormat=Structure With Time  SampleTime=-1
  travTimeL9 : ToWorkspace  VariableName=travTimeL9  SaveFormat=Structure With Time  SampleTime=-1
  vacanInS1 : ToWorkspace  VariableName=vacanInS1  SaveFormat=Structure With Time  SampleTime=-1
  vacanInS10 : ToWorkspace  VariableName=vacanInS10  SaveFormat=Structure With Time  SampleTime=-1
  vacanInS11 : ToWorkspace  VariableName=vacanInS11  SaveFormat=Structure With Time  SampleTime=-1
  vacanInS12 : ToWorkspace  VariableName=vacanInS12  SaveFormat=Structure With Time  SampleTime=-1
  vacanInS13 : ToWorkspace  VariableName=vacanInS13  SaveFormat=Structure With Time  SampleTime=-1
  vacanInS14 : ToWorkspace  VariableName=vacanInS14  SaveFormat=Structure With Time  SampleTime=-1
  vacanInS15 : ToWorkspace  VariableName=vacanInS15  SaveFormat=Structure With Time  SampleTime=-1
  vacanInS16 : ToWorkspace  VariableName=vacanInS16  SaveFormat=Structure With Time  SampleTime=-1
  vacanInS17 : ToWorkspace  VariableName=vacanInS17  SaveFormat=Structure With Time  SampleTime=-1
  vacanInS18 : ToWorkspace  VariableName=vacanInS18  SaveFormat=Structure With Time  SampleTime=-1
  vacanInS2 : ToWorkspace  VariableName=vacanInS2  SaveFormat=Structure With Time  SampleTime=-1
  vacanInS3 : ToWorkspace  VariableName=vacanInS3  SaveFormat=Structure With Time  SampleTime=-1
  vacanInS4 : ToWorkspace  VariableName=vacanInS4  SaveFormat=Structure With Time  SampleTime=-1
  vacanInS5 : ToWorkspace  VariableName=vacanInS5  SaveFormat=Structure With Time  SampleTime=-1
  vacanInS6 : ToWorkspace  VariableName=vacanInS6  SaveFormat=Structure With Time  SampleTime=-1
  vacanInS7 : ToWorkspace  VariableName=vacanInS7  SaveFormat=Structure With Time  SampleTime=-1
  vacanInS8 : ToWorkspace  VariableName=vacanInS8  SaveFormat=Structure With Time  SampleTime=-1
  vacanInS9 : ToWorkspace  VariableName=vacanInS9  SaveFormat=Structure With Time  SampleTime=-1
  wires:
  Constant2/1 -> T2E7/1
  Get Attribute2/1 -> idInit/1
  bus1IntergenTime/1 -> bus1Generator/1
  T2E7/1 -> Set Attribute/1
  Subsystem/1(schedTime) -> Set Attribute8/1
  Event Filter/1 -> Subsystem/1(ID)
  From Workspace1/1 -> T2E15/1
  Get Attribute4/1 -> idNxtNormalBus/1, Event Filter/1
  Get Attribute/1 -> Add/2, idAfterCycle/1
  Get Attribute10/1 -> idBus4SA/1
  Get Attribute11/1 -> idBus3SA/1
  Get Attribute12/1 -> idBus2SA/1
  Get Attribute13/1 -> idBus1SA/1
  Event Filter2/1 -> Subsystem3/1(crnSched)
  Event Filter3/1 -> Subsystem3/2(time)
  T2E1/1 -> Set Attribute8/2
  Clock/1 -> T2E1/1
  Get Attribute3/3 -> timeArr/1, Event Filter3/1
  T2E15/1 -> Subsystem/2(tTable)
  Subsystem3/1(tHoldCrnBus) -> HoldMultiBus/1, tHold/1
  Get Attribute3/1 -> Event Filter2/1, timeScheduled/1
  Get Attribute3/2 -> busIDOut/1
  T2E4/1 -> Set Attribute/3, Set Attribute/2
  maxCapBus1/1 -> T2E4/1
  tBoardPerPax/1 -> T2E10/1
  T2E10/1 -> Set Attribute/4
  Constant1/1 -> T2E9/1
  bus2IntergenTime/1 -> bus2Generator/1
  T2E9/1 -> Set Attribute3/1
  T2E8/1 -> Set Attribute3/3, Set Attribute3/2
  maxCapBus2/1 -> T2E8/1
  tBoardPerPax1/1 -> T2E5/1
  T2E5/1 -> Set Attribute3/4
  Constant3/1 -> T2E16/1
  bus3IntergenTime/1 -> bus3Generator/1
  T2E16/1 -> Set Attribute4/1
  T2E13/1 -> Set Attribute4/3, Set Attribute4/2
  maxCapBus3/1 -> T2E13/1
  tBoardPerPax2/1 -> T2E12/1
  T2E12/1 -> Set Attribute4/4
  Constant4/1 -> T2E19/1
  bus4IntergenTime/1 -> bus4Generator/1
  T2E19/1 -> Set Attribute5/1
  T2E17/1 -> Set Attribute5/3, Set Attribute5/2
  maxCapBus4/1 -> T2E17/1
  tBoardPerPax3/1 -> T2E14/1
  T2E14/1 -> Set Attribute5/4
  delayL1/1 -> Rounding/1
  inTransitLinkL1/1(idBusOutLink) -> idBusOutL1/1
  tTravL1/1 -> T2E20/1
  T2E20/1 -> inTransitLinkL1/2(theoTravTime), travTimeL1/1
  T2E21/1 -> randDelayL1/1, inTransitLinkL1/1(xtraDelay)
  Rounding/1 -> T2E21/1
  ratePaxArrS1/1 -> atStopS1/1(paxDemandRate)
  ratePaxAlightS1/1 -> atStopS1/2(paxAlightRate)
  atStopS1/1(accPaxAlight) -> rawPaxAlightS1/1
  atStopS1/2(accPaxDemand) -> rawPaxDemandS1/1
  atStopS1/3(crnVacancy) -> vacanInS1/1
  atStopS1/4(paxAlight) -> paxAlightS1/1
  atStopS1/5(paxDemand) -> paxDemandS1/1
  atStopS1/6(busIDAfterPaxCal) -> idBusArrS1/1
  atStopS1/7(newVacancy) -> newVacanS1/1
  atStopS1/8(paxBoard) -> paxBoardS1/1
  atStopS1/9(paxRemain) -> paxRemainS1/1
  atStopS1/10(paxWait) -> paxWaitS1/1
  atStopS1/11(intgPaxArr) -> intgPaxArrS1/1
  atStopS1/12(intgPaxAlight) -> intgPaxAlightS1/1
  atStopS1/13(idBusLeave) -> idBusOutS1/1
  delayL2/1 -> Rounding1/1
  inTransitLinkL2/1(idBusOutLink) -> idBusOutL2/1
  tTravL2/1 -> T2E22/1
  T2E22/1 -> inTransitLinkL2/2(theoTravTime), travTimeL2/1
  T2E23/1 -> inTransitLinkL2/1(xtraDelay), randDelayL2/1
  Rounding1/1 -> T2E23/1
  ratePaxArrS2/1 -> atStopS2/1(paxDemandRate)
  ratePaxAlightS2/1 -> atStopS2/2(paxAlightRate)
  atStopS2/1(accPaxAlight) -> rawPaxAlightS2/1
  atStopS2/2(accPaxDemand) -> rawPaxDemandS2/1
  atStopS2/3(crnVacancy) -> vacanInS2/1
  atStopS2/4(paxAlight) -> paxAlightS2/1
  atStopS2/5(paxDemand) -> paxDemandS2/1
  atStopS2/6(busIDAfterPaxCal) -> idBusArrS2/1
  atStopS2/7(newVacancy) -> newVacanS2/1
  atStopS2/8(paxBoard) -> paxBoardS2/1
  atStopS2/9(paxRemain) -> paxRemainS2/1
  atStopS2/10(paxWait) -> paxWaitS2/1
  atStopS2/11(intgPaxArr) -> intgPaxArrS2/1
  atStopS2/12(intgPaxAlight) -> intgPaxAlightS2/1
  atStopS2/13(idBusLeave) -> idBusOutS2/1
  delayL3/1 -> Rounding2/1
  inTransitLinkL3/1(idBusOutLink) -> idBusOutL3/1
  tTravL3/1 -> T2E24/1
  T2E24/1 -> inTransitLinkL3/2(theoTravTime), travTimeL3/1
  T2E25/1 -> inTransitLinkL3/1(xtraDelay), randDelayL3/1
  Rounding2/1 -> T2E25/1
  ratePaxArrS3/1 -> atStopS3/1(paxDemandRate)
  ratePaxAlightS3/1 -> atStopS3/2(paxAlightRate)
  atStopS3/1(accPaxAlight) -> rawPaxAlightS3/1
  atStopS3/2(accPaxDemand) -> rawPaxDemandS3/1
  atStopS3/3(crnVacancy) -> vacanInS3/1
  atStopS3/4(paxAlight) -> paxAlightS3/1
  atStopS3/5(paxDemand) -> paxDemandS3/1
  atStopS3/6(busIDAfterPaxCal) -> idBusArrS3/1
  atStopS3/7(newVacancy) -> newVacanS3/1
  atStopS3/8(paxBoard) -> paxBoardS3/1
  atStopS3/9(paxRemain) -> paxRemainS3/1
  atStopS3/10(paxWait) -> paxWaitS3/1
  atStopS3/11(intgPaxArr) -> intgPaxArrS3/1
  atStopS3/12(intgPaxAlight) -> intgPaxAlightS3/1
  atStopS3/13(idBusLeave) -> idBusOutS3/1
  delayL4/1 -> Rounding3/1
  inTransitLinkL4/1(idBusOutLink) -> idBusOutL4/1
  tTravL4/1 -> T2E26/1
  T2E26/1 -> inTransitLinkL4/2(theoTravTime), travTimeL4/1
  T2E27/1 -> inTransitLinkL4/1(xtraDelay), randDelayL4/1
  Rounding3/1 -> T2E27/1
  ratePaxArrS4/1 -> atStopS4/1(paxDemandRate)
  ratePaxAlightS4/1 -> atStopS4/2(paxAlightRate)
  atStopS4/1(accPaxAlight) -> rawPaxAlightS4/1
  atStopS4/2(accPaxDemand) -> rawPaxDemandS4/1
  atStopS4/3(crnVacancy) -> vacanInS4/1
  atStopS4/4(paxAlight) -> paxAlightS4/1
  atStopS4/5(paxDemand) -> paxDemandS4/1
  atStopS4/6(busIDAfterPaxCal) -> idBusArrS4/1
  atStopS4/7(newVacancy) -> newVacanS4/1
  atStopS4/8(paxBoard) -> paxBoardS4/1
  atStopS4/9(paxRemain) -> paxRemainS4/1
  atStopS4/10(paxWait) -> paxWaitS4/1
  atStopS4/11(intgPaxArr) -> intgPaxArrS4/1
  atStopS4/12(intgPaxAlight) -> intgPaxAlightS4/1
  atStopS4/13(idBusLeave) -> idBusOutS4/1
  Get Attribute5/1 -> idBusOutChkPntEndCycle/1
  delayL5/1 -> Rounding4/1
  inTransitLinkL5/1(idBusOutLink) -> idBusOutL5/1
  tTravL5/1 -> T2E30/1
  T2E30/1 -> travTimeL5/1, inTransitLinkL5/2(theoTravTime)
  T2E31/1 -> randDelayL5/1, inTransitLinkL5/1(xtraDelay)
  Rounding4/1 -> T2E31/1
  ratePaxArrS5/1 -> atStopS5/1(paxDemandRate)
  ratePaxAlightS5/1 -> atStopS5/2(paxAlightRate)
  atStopS5/1(accPaxAlight) -> rawPaxAlightS5/1
  atStopS5/2(accPaxDemand) -> rawPaxDemandS5/1
  atStopS5/3(crnVacancy) -> vacanInS5/1
  atStopS5/4(paxAlight) -> paxAlightS5/1
  atStopS5/5(paxDemand) -> paxDemandS5/1
  atStopS5/6(busIDAfterPaxCal) -> idBusArrAfterCPS5/1
  atStopS5/7(newVacancy) -> newVacanS5/1
  atStopS5/8(paxBoard) -> paxBoardS5/1
  atStopS5/9(paxRemain) -> paxRemainS5/1
  atStopS5/10(paxWait) -> paxWaitS5/1
  atStopS5/11(intgPaxArr) -> intgPaxArrS5/1
  atStopS5/12(intgPaxAlight) -> intgPaxAlightS5/1
  atStopS5/13(idBusLeave) -> idBusOutS5/1
  delayL6/1 -> Rounding5/1
  inTransitLinkL6/1(idBusOutLink) -> idBusOutL6/1
  tTravL6/1 -> T2E34/1
  T2E34/1 -> travTimeL6/1, inTransitLinkL6/2(theoTravTime)
  T2E35/1 -> randDelayL6/1, inTransitLinkL6/1(xtraDelay)
  Rounding5/1 -> T2E35/1
  ratePaxArrS6/1 -> atStopS6/1(paxDemandRate)
  ratePaxAlightS6/1 -> atStopS6/2(paxAlightRate)
  atStopS6/1(accPaxAlight) -> rawPaxAlightS6/1
  atStopS6/2(accPaxDemand) -> rawPaxDemandS6/1
  atStopS6/3(crnVacancy) -> vacanInS6/1
  atStopS6/4(paxAlight) -> paxAlightS6/1
  atStopS6/5(paxDemand) -> paxDemandS6/1
  atStopS6/6(busIDAfterPaxCal) -> idBusArrS6/1
  atStopS6/7(newVacancy) -> newVacanS6/1
  atStopS6/8(paxBoard) -> paxBoardS6/1
  atStopS6/9(paxRemain) -> paxRemainS6/1
  atStopS6/10(paxWait) -> paxWaitS6/1
  atStopS6/11(intgPaxArr) -> intgPaxArrS6/1
  atStopS6/12(intgPaxAlight) -> intgPaxAlightS6/1
  atStopS6/13(idBusLeave) -> idBusOutS6/1
  delayL7/1 -> Rounding6/1
  inTransitLinkL7/1(idBusOutLink) -> idBusOutL7/1
  tTravL7/1 -> T2E36/1
  T2E36/1 -> travTimeL7/1, inTransitLinkL7/2(theoTravTime)
  T2E37/1 -> randDelayL7/1, inTransitLinkL7/1(xtraDelay)
  Rounding6/1 -> T2E37/1
  ratePaxArrS7/1 -> atStopS7/1(paxDemandRate)
  ratePaxAlightS7/1 -> atStopS7/2(paxAlightRate)
  atStopS7/1(accPaxAlight) -> rawPaxAlightS7/1
  atStopS7/2(accPaxDemand) -> rawPaxDemandS7/1
  atStopS7/3(crnVacancy) -> vacanInS7/1
  atStopS7/4(paxAlight) -> paxAlightS7/1
  atStopS7/5(paxDemand) -> paxDemandS7/1
  atStopS7/6(busIDAfterPaxCal) -> idBusArrS7/1
  atStopS7/7(newVacancy) -> newVacanS7/1
  atStopS7/8(paxBoard) -> paxBoardS7/1
  atStopS7/9(paxRemain) -> paxRemainS7/1
  atStopS7/10(paxWait) -> paxWaitS7/1
  atStopS7/11(intgPaxArr) -> intgPaxArrS7/1
  atStopS7/12(intgPaxAlight) -> intgPaxAlightS7/1
  atStopS7/13(idBusLeave) -> idBusOutS7/1
  delayL8/1 -> Rounding7/1
  inTransitLinkL8/1(idBusOutLink) -> idBusOutL8/1
  tTravL8/1 -> T2E38/1
  T2E38/1 -> travTimeL8/1, inTransitLinkL8/2(theoTravTime)
  T2E39/1 -> randDelayL8/1, inTransitLinkL8/1(xtraDelay)
  Rounding7/1 -> T2E39/1
  ratePaxArrS8/1 -> atStopS8/1(paxDemandRate)
  ratePaxAlightS8/1 -> atStopS8/2(paxAlightRate)
  atStopS8/1(accPaxAlight) -> rawPaxAlightS8/1
  atStopS8/2(accPaxDemand) -> rawPaxDemandS8/1
  atStopS8/3(crnVacancy) -> vacanInS8/1
  atStopS8/4(paxAlight) -> paxAlightS8/1
  atStopS8/5(paxDemand) -> paxDemandS8/1
  atStopS8/6(busIDAfterPaxCal) -> idBusArrS8/1
  atStopS8/7(newVacancy) -> newVacanS8/1
  atStopS8/8(paxBoard) -> paxBoardS8/1
  atStopS8/9(paxRemain) -> paxRemainS8/1
  atStopS8/10(paxWait) -> paxWaitS8/1
  atStopS8/11(intgPaxArr) -> intgPaxArrS8/1
  atStopS8/12(intgPaxAlight) -> intgPaxAlightS8/1
  atStopS8/13(idBusLeave) -> idBusOutS8/1
  delayL9/1 -> Rounding8/1
  inTransitLinkL9/1(idBusOutLink) -> idBusOutL9/1
  tTravL9/1 -> T2E40/1
  T2E40/1 -> travTimeL9/1, inTransitLinkL9/2(theoTravTime)
  T2E41/1 -> randDelayL9/1, inTransitLinkL9/1(xtraDelay)
  Rounding8/1 -> T2E41/1
  ratePaxArrS9/1 -> atStopS9/1(paxDemandRate)
  ratePaxAlightS9/1 -> atStopS9/2(paxAlightRate)
  atStopS9/1(accPaxAlight) -> rawPaxAlightS9/1
  atStopS9/2(accPaxDemand) -> rawPaxDemandS9/1
  atStopS9/3(crnVacancy) -> vacanInS9/1
  atStopS9/4(paxAlight) -> paxAlightS9/1
  atStopS9/5(paxDemand) -> paxDemandS9/1
  atStopS9/6(busIDAfterPaxCal) -> idBusArrS9/1
  atStopS9/7(newVacancy) -> newVacanS9/1
  atStopS9/8(paxBoard) -> paxBoardS9/1
  atStopS9/9(paxRemain) -> paxRemainS9/1
  atStopS9/10(paxWait) -> paxWaitS9/1
  atStopS9/11(intgPaxArr) -> intgPaxArrS9/1
  atStopS9/12(intgPaxAlight) -> intgPaxAlightS9/1
  atStopS9/13(idBusLeave) -> idBusOutS9/1
  delayL10/1 -> Rounding9/1
  inTransitLinkL10/1(idBusOutLink) -> idBusOutL10/1
  tTravL10/1 -> T2E42/1
  T2E42/1 -> inTransitLinkL10/2(theoTravTime), travTimeL10/1
  T2E43/1 -> inTransitLinkL10/1(xtraDelay), randDelayL10/1
  Rounding9/1 -> T2E43/1
  ratePaxArrS10/1 -> atStopS10/1(paxDemandRate)
  ratePaxAlightS10/1 -> atStopS10/2(paxAlightRate)
  atStopS10/1(accPaxAlight) -> rawPaxAlightS10/1
  atStopS10/2(accPaxDemand) -> rawPaxDemandS10/1
  atStopS10/3(crnVacancy) -> vacanInS10/1
  atStopS10/4(paxAlight) -> paxAlightS10/1
  atStopS10/5(paxDemand) -> paxDemandS10/1
  atStopS10/6(busIDAfterPaxCal) -> idBusArrS10/1
  atStopS10/7(newVacancy) -> newVacanS10/1
  atStopS10/8(paxBoard) -> paxBoardS10/1
  atStopS10/9(paxRemain) -> paxRemainS10/1
  atStopS10/10(paxWait) -> paxWaitS10/1
  atStopS10/11(intgPaxArr) -> intgPaxArrS10/1
  atStopS10/12(intgPaxAlight) -> intgPaxAlightS10/1
  atStopS10/13(idBusLeave) -> idBusOutS10/1
  delayL11/1 -> Rounding10/1
  inTransitLinkL11/1(idBusOutLink) -> idBusOutL11/1
  tTravL11/1 -> T2E44/1
  T2E44/1 -> travTimeL11/1, inTransitLinkL11/2(theoTravTime)
  T2E45/1 -> randDelayL11/1, inTransitLinkL11/1(xtraDelay)
  Rounding10/1 -> T2E45/1
  ratePaxArrS11/1 -> atStopS11/1(paxDemandRate)
  ratePaxAlightS11/1 -> atStopS11/2(paxAlightRate)
  atStopS11/1(accPaxAlight) -> rawPaxAlightS11/1
  atStopS11/2(accPaxDemand) -> rawPaxDemandS11/1
  atStopS11/3(crnVacancy) -> vacanInS11/1
  atStopS11/4(paxAlight) -> paxAlightS11/1
  atStopS11/5(paxDemand) -> paxDemandS11/1
  atStopS11/6(busIDAfterPaxCal) -> idBusArrAfterCPS11/1
  atStopS11/7(newVacancy) -> newVacanS11/1
  atStopS11/8(paxBoard) -> paxBoardS11/1
  atStopS11/9(paxRemain) -> paxRemainS11/1
  atStopS11/10(paxWait) -> paxWaitS11/1
  atStopS11/11(intgPaxArr) -> intgPaxArrS11/1
  atStopS11/12(intgPaxAlight) -> intgPaxAlightS11/1
  atStopS11/13(idBusLeave) -> idBusOutS11/1
  Get Attribute7/1 -> idBusArrS11/1
  delayL12/1 -> Rounding11/1
  inTransitLinkL12/1(idBusOutLink) -> idBusOutL12/1
  tTravL12/1 -> T2E48/1
  T2E48/1 -> travTimeL12/1, inTransitLinkL12/2(theoTravTime)
  T2E49/1 -> randDelayL12/1, inTransitLinkL12/1(xtraDelay)
  Rounding11/1 -> T2E49/1
  ratePaxArrS12/1 -> atStopS12/1(paxDemandRate)
  ratePaxAlightS12/1 -> atStopS12/2(paxAlightRate)
  atStopS12/1(accPaxAlight) -> rawPaxAlightS12/1
  atStopS12/2(accPaxDemand) -> rawPaxDemandS12/1
  atStopS12/3(crnVacancy) -> vacanInS12/1
  atStopS12/4(paxAlight) -> paxAlightS12/1
  atStopS12/5(paxDemand) -> paxDemandS12/1
  atStopS12/6(busIDAfterPaxCal) -> idBusArrS12/1
  atStopS12/7(newVacancy) -> newVacanS12/1
  atStopS12/8(paxBoard) -> paxBoardS12/1
  atStopS12/9(paxRemain) -> paxRemainS12/1
  atStopS12/10(paxWait) -> paxWaitS12/1
  atStopS12/11(intgPaxArr) -> intgPaxArrS12/1
  atStopS12/12(intgPaxAlight) -> intgPaxAlightS12/1
  atStopS12/13(idBusLeave) -> idBusOutS12/1
  delayL13/1 -> Rounding12/1
  inTransitLinkL13/1(idBusOutLink) -> idBusOutL13/1
  tTravL13/1 -> T2E50/1
  T2E50/1 -> travTimeL13/1, inTransitLinkL13/2(theoTravTime)
  T2E51/1 -> randDelayL13/1, inTransitLinkL13/1(xtraDelay)
  Rounding12/1 -> T2E51/1
  ratePaxArrS13/1 -> atStopS13/1(paxDemandRate)
  ratePaxAlightS13/1 -> atStopS13/2(paxAlightRate)
  atStopS13/1(accPaxAlight) -> rawPaxAlightS13/1
  atStopS13/2(accPaxDemand) -> rawPaxDemandS13/1
  atStopS13/3(crnVacancy) -> vacanInS13/1
  atStopS13/4(paxAlight) -> paxAlightS13/1
  atStopS13/5(paxDemand) -> paxDemandS13/1
  atStopS13/6(busIDAfterPaxCal) -> idBusArrS13/1
  atStopS13/7(newVacancy) -> newVacanS13/1
  atStopS13/8(paxBoard) -> paxBoardS13/1
  atStopS13/9(paxRemain) -> paxRemainS13/1
  atStopS13/10(paxWait) -> paxWaitS13/1
  atStopS13/11(intgPaxArr) -> intgPaxArrS13/1
  atStopS13/12(intgPaxAlight) -> intgPaxAlightS13/1
  atStopS13/13(idBusLeave) -> idBusOutS13/1
  delayL14/1 -> Rounding13/1
  inTransitLinkL14/1(idBusOutLink) -> idBusOutL14/1
  tTravL14/1 -> T2E52/1
  T2E52/1 -> inTransitLinkL14/2(theoTravTime), travTimeL14/1
  T2E53/1 -> inTransitLinkL14/1(xtraDelay), randDelayL14/1
  Rounding13/1 -> T2E53/1
  ratePaxArrS14/1 -> atStopS14/1(paxDemandRate)
  ratePaxAlightS14/1 -> atStopS14/2(paxAlightRate)
  atStopS14/1(accPaxAlight) -> rawPaxAlightS14/1
  atStopS14/2(accPaxDemand) -> rawPaxDemandS14/1
  atStopS14/3(crnVacancy) -> vacanInS14/1
  atStopS14/4(paxAlight) -> paxAlightS14/1
  atStopS14/5(paxDemand) -> paxDemandS14/1
  atStopS14/6(busIDAfterPaxCal) -> idBusArrAfterCPS14/1
  atStopS14/7(newVacancy) -> newVacanS14/1
  atStopS14/8(paxBoard) -> paxBoardS14/1
  atStopS14/9(paxRemain) -> paxRemainS14/1
  atStopS14/10(paxWait) -> paxWaitS14/1
  atStopS14/11(intgPaxArr) -> intgPaxArrS14/1
  atStopS14/12(intgPaxAlight) -> intgPaxAlightS14/1
  atStopS14/13(idBusLeave) -> idBusOutS14/1
  Get Attribute8/1 -> idBusArrS14/1
  delayL15/1 -> Rounding14/1
  inTransitLinkL15/1(idBusOutLink) -> idBusOutL15/1
  tTravL15/1 -> T2E56/1
  T2E56/1 -> inTransitLinkL15/2(theoTravTime), travTimeL15/1
  T2E57/1 -> inTransitLinkL15/1(xtraDelay), randDelayL15/1
  Rounding14/1 -> T2E57/1
  ratePaxArrS15/1 -> atStopS15/1(paxDemandRate)
  ratePaxAlightS15/1 -> atStopS15/2(paxAlightRate)
  atStopS15/1(accPaxAlight) -> rawPaxAlightS15/1
  atStopS15/2(accPaxDemand) -> rawPaxDemandS15/1
  atStopS15/3(crnVacancy) -> vacanInS15/1
  atStopS15/4(paxAlight) -> paxAlightS15/1
  atStopS15/5(paxDemand) -> paxDemandS15/1
  atStopS15/6(busIDAfterPaxCal) -> idBusArrS15/1
  atStopS15/7(newVacancy) -> newVacanS15/1
  atStopS15/8(paxBoard) -> paxBoardS15/1
  atStopS15/9(paxRemain) -> paxRemainS15/1
  atStopS15/10(paxWait) -> paxWaitS15/1
  atStopS15/11(intgPaxArr) -> intgPaxArrS15/1
  atStopS15/12(intgPaxAlight) -> intgPaxAlightS15/1
  atStopS15/13(idBusLeave) -> idBusOutS15/1
  delayL16/1 -> Rounding15/1
  inTransitLinkL16/1(idBusOutLink) -> idBusOutL16/1
  tTravL16/1 -> T2E58/1
  T2E58/1 -> travTimeL16/1, inTransitLinkL16/2(theoTravTime)
  T2E59/1 -> randDelayL16/1, inTransitLinkL16/1(xtraDelay)
  Rounding15/1 -> T2E59/1
  ratePaxArrS16/1 -> atStopS16/1(paxDemandRate)
  ratePaxAlightS16/1 -> atStopS16/2(paxAlightRate)
  atStopS16/1(accPaxAlight) -> rawPaxAlightS16/1
  atStopS16/2(accPaxDemand) -> rawPaxDemandS16/1
  atStopS16/3(crnVacancy) -> vacanInS16/1
  atStopS16/4(paxAlight) -> paxAlightS16/1
  atStopS16/5(paxDemand) -> paxDemandS16/1
  atStopS16/6(busIDAfterPaxCal) -> idBusArrS16/1
  atStopS16/7(newVacancy) -> newVacanS16/1
  atStopS16/8(paxBoard) -> paxBoardS16/1
  atStopS16/9(paxRemain) -> paxRemainS16/1
  atStopS16/10(paxWait) -> paxWaitS16/1
  atStopS16/11(intgPaxArr) -> intgPaxArrS16/1
  atStopS16/12(intgPaxAlight) -> intgPaxAlightS16/1
  atStopS16/13(idBusLeave) -> idBusOutS16/1
  delayL17/1 -> Rounding16/1
  inTransitLinkL17/1(idBusOutLink) -> idBusOutL17/1
  tTravL17/1 -> T2E61/1
  T2E61/1 -> inTransitLinkL17/2(theoTravTime), travTimeL17/1
  T2E62/1 -> inTransitLinkL17/1(xtraDelay), randDelayL17/1
  Rounding16/1 -> T2E62/1
  ratePaxArrS17/1 -> atStopS17/1(paxDemandRate)
  ratePaxAlightS17/1 -> atStopS17/2(paxAlightRate)
  atStopS17/1(accPaxAlight) -> rawPaxAlightS17/1
  atStopS17/2(accPaxDemand) -> rawPaxDemandS17/1
  atStopS17/3(crnVacancy) -> vacanInS17/1
  atStopS17/4(paxAlight) -> paxAlightS17/1
  atStopS17/5(paxDemand) -> paxDemandS17/1
  atStopS17/6(busIDAfterPaxCal) -> idBusArrS17/1
  atStopS17/7(newVacancy) -> newVacanS17/1
  atStopS17/8(paxBoard) -> paxBoardS17/1
  atStopS17/9(paxRemain) -> paxRemainS17/1
  atStopS17/10(paxWait) -> paxWaitS17/1
  atStopS17/11(intgPaxArr) -> intgPaxArrS17/1
  atStopS17/12(intgPaxAlight) -> intgPaxAlightS17/1
  atStopS17/13(idBusLeave) -> idBusOutS17/1
  delayL18/1 -> Rounding17/1
  inTransitLinkL18/1(idBusOutLink) -> idBusOutL18/1
  tTravL18/1 -> T2E63/1
  T2E63/1 -> travTimeL18/1, inTransitLinkL18/2(theoTravTime)
  T2E64/1 -> randDelayL18/1, inTransitLinkL18/1(xtraDelay)
  Rounding17/1 -> T2E64/1
  ratePaxArrS18/1 -> atStopS18/1(paxDemandRate)
  ratePaxAlightS18/1 -> atStopS18/2(paxAlightRate)
  atStopS18/1(accPaxAlight) -> rawPaxAlightS18/1
  atStopS18/2(accPaxDemand) -> rawPaxDemandS18/1
  atStopS18/3(crnVacancy) -> vacanInS18/1
  atStopS18/4(paxAlight) -> paxAlightS18/1
  atStopS18/5(paxDemand) -> paxDemandS18/1
  atStopS18/6(busIDAfterPaxCal) -> idBusArrS18/1
  atStopS18/7(newVacancy) -> newVacanS18/1
  atStopS18/8(paxBoard) -> paxBoardS18/1
  atStopS18/9(paxRemain) -> paxRemainS18/1
  atStopS18/10(paxWait) -> paxWaitS18/1
  atStopS18/11(intgPaxArr) -> intgPaxArrS18/1
  atStopS18/12(intgPaxAlight) -> intgPaxAlightS18/1
  atStopS18/13(idBusLeave) -> idBusOutS18/1
  Get Attribute6/1 -> idBusArrS5/1
  From Workspace2/1 -> chkSchedTimeNormalBusAtCP2/1(tTableChkPnt)
  Get Attribute19/1 -> idBusOutChkPntS5/1
  From Workspace3/1 -> chkSchedTimeNormalBusAtCP3/1(tTableChkPnt)
  Get Attribute22/1 -> idBusOutChkPntS11/1
  holdBusAtCP2/1(idB4CP) -> idB4CP2/1
  holdBusAtCP2/2(tSchedCP) -> tSchedCP2/1
  holdBusAtCP2/3(tHoldCP) -> tHoldCP2/1
  From Workspace4/1 -> chkSchedTimeNormalBusAtCP4/1(tTableChkPnt)
  Get Attribute17/1 -> idBusOutChkPntS14/1
  holdBusAtCP3/1(idB4CP) -> idB4CP3/1
  holdBusAtCP3/2(tSchedCP) -> tSchedCP3/1
  holdBusAtCP3/3(tHoldCP) -> tHoldCP3/1
  holdBusAtCP4/1(idB4CP) -> idB4CP4/1
  holdBusAtCP4/2(tSchedCP) -> tSchedCP4/1
  holdBusAtCP4/3(tHoldCP) -> tHoldCP4/1
  Constant/1 -> Add/1
  Add/1 -> Set Attribute9/1
  connections:
  bus1Generator/RConn1 -- dummy Server/LConn1
  dummy Server/RConn1 -- Set Attribute/LConn1
  Set Attribute/RConn1 -- Get Attribute13/LConn1
  atStopS1/LConn1 -- Get Attribute2/RConn1
  Path Combiner/RConn1 -- FIFO Queue8/LConn1
  Get Attribute12/LConn1 -- Set Attribute3/RConn1
  Set Attribute4/RConn1 -- Get Attribute11/LConn1
  Set Attribute5/RConn1 -- Get Attribute10/LConn1
  Get Attribute/RConn1 -- FIFO Queue2/LConn1
  Set Attribute8/RConn1 -- Get Attribute3/LConn1
  FIFO Queue6/RConn1 -- Set Attribute8/LConn1
  Get Attribute3/RConn1 -- dummyServer/LConn1
  Get Attribute4/RConn1 -- FIFO Queue6/LConn1
  Get Attribute12/RConn1 -- FIFO Queue16/LConn1
  Get Attribute10/RConn1 -- FIFO Queue14/LConn1
  Get Attribute11/RConn1 -- FIFO Queue15/LConn1
  Get Attribute13/RConn1 -- FIFO Queue17/LConn1
  HoldMultiBus/RConn1 -- Get Attribute5/LConn1
  Get Attribute5/RConn1 -- FIFO Queue13/LConn1
  FIFO Queue14/RConn1 -- Path Combiner/LConn4
  FIFO Queue15/RConn1 -- Path Combiner/LConn3
  FIFO Queue16/RConn1 -- Path Combiner/LConn2
  FIFO Queue17/RConn1 -- Path Combiner/LConn1
  dummy Server1/RConn1 -- Set Attribute3/LConn1
  bus2Generator/RConn1 -- dummy Server1/LConn1
  dummy Server2/RConn1 -- Set Attribute4/LConn1
  bus3Generator/RConn1 -- dummy Server2/LConn1
  dummy Server3/RConn1 -- Set Attribute5/LConn1
  bus4Generator/RConn1 -- dummy Server3/LConn1
  atStopS1/RConn1 -- inTransitLinkL1/LConn1
  inTransitLinkL2/LConn1 -- atStopS2/RConn1
  atStopS2/LConn1 -- inTransitLinkL1/RConn1
  inTransitLinkL2/RConn1 -- atStopS3/LConn1
  inTransitLinkL3/LConn1 -- atStopS3/RConn1
  inTransitLinkL4/LConn1 -- atStopS4/RConn1
  inTransitLinkL3/RConn1 -- atStopS4/LConn1
  dummyServer/RConn1 -- HoldMultiBus/LConn1
  FIFO Queue13/RConn1 -- Path Combiner/LConn5
  FIFO Queue8/RConn1 -- Get Attribute2/LConn1
  inTransitLinkL5/LConn1 -- atStopS5/RConn1
  Get Attribute6/LConn1 -- inTransitLinkL4/RConn1
  inTransitLinkL5/RConn1 -- atStopS6/LConn1
  inTransitLinkL6/LConn1 -- atStopS6/RConn1
  inTransitLinkL7/LConn1 -- atStopS7/RConn1
  inTransitLinkL6/RConn1 -- atStopS7/LConn1
  inTransitLinkL8/LConn1 -- atStopS8/RConn1
  inTransitLinkL7/RConn1 -- atStopS8/LConn1
  inTransitLinkL9/LConn1 -- atStopS9/RConn1
  inTransitLinkL8/RConn1 -- atStopS9/LConn1
  inTransitLinkL9/RConn1 -- atStopS10/LConn1
  inTransitLinkL10/LConn1 -- atStopS10/RConn1
  inTransitLinkL10/RConn1 -- Get Attribute7/LConn1
  inTransitLinkL11/LConn1 -- atStopS11/RConn1
  FIFO Queue4/RConn1 -- chkSchedTimeNormalBusAtCP3/LConn1
  Get Attribute7/RConn1 -- FIFO Queue4/LConn1
  inTransitLinkL11/RConn1 -- atStopS12/LConn1
  inTransitLinkL12/LConn1 -- atStopS12/RConn1
  inTransitLinkL12/RConn1 -- atStopS13/LConn1
  inTransitLinkL13/LConn1 -- atStopS13/RConn1
  inTransitLinkL13/RConn1 -- Get Attribute8/LConn1
  inTransitLinkL14/LConn1 -- atStopS14/RConn1
  Get Attribute8/RConn1 -- FIFO Queue5/LConn1
  FIFO Queue5/RConn1 -- chkSchedTimeNormalBusAtCP4/LConn1
  inTransitLinkL14/RConn1 -- atStopS15/LConn1
  inTransitLinkL15/LConn1 -- atStopS15/RConn1
  inTransitLinkL16/LConn1 -- atStopS16/RConn1
  inTransitLinkL15/RConn1 -- atStopS16/LConn1
  inTransitLinkL17/LConn1 -- atStopS17/RConn1
  inTransitLinkL16/RConn1 -- atStopS17/LConn1
  inTransitLinkL18/LConn1 -- atStopS18/RConn1
  inTransitLinkL17/RConn1 -- atStopS18/LConn1
  inTransitLinkL18/RConn1 -- FIFO Queue10/LConn1
  FIFO Queue3/RConn1 -- chkSchedTimeNormalBusAtCP2/LConn1
  Get Attribute6/RConn1 -- FIFO Queue3/LConn1
  Get Attribute19/RConn1 -- atStopS5/LConn1
  atStopS11/LConn1 -- Get Attribute22/RConn1
  chkSchedTimeNormalBusAtCP3/RConn1 -- holdBusAtCP3/LConn1
  holdBusAtCP3/RConn1 -- Get Attribute22/LConn1
  chkSchedTimeNormalBusAtCP2/RConn1 -- holdBusAtCP2/LConn1
  holdBusAtCP2/RConn1 -- Get Attribute19/LConn1
  holdBusAtCP4/RConn1 -- Get Attribute17/LConn1
  atStopS14/LConn1 -- Get Attribute17/RConn1
  chkSchedTimeNormalBusAtCP4/RConn1 -- holdBusAtCP4/LConn1
  Get Attribute/LConn1 -- FIFO Queue10/RConn1
  Set Attribute9/RConn1 -- Get Attribute4/LConn1
  FIFO Queue2/RConn1 -- Set Attribute9/LConn1
